simulink model "newFS_safetyTests"  (R2019a)
settings: Solver=FixedStepAuto  StartTime=0.0  StopTime=70  FixedStep=0.01  RelTol=1e-3
libraries: simulink x2, autolibshared x2, vehdynlibsteering x2, autolibutils x2, eeGeneralControl x1
settings Model: Creator=ckreienk  LastModifiedBy=ckreienk

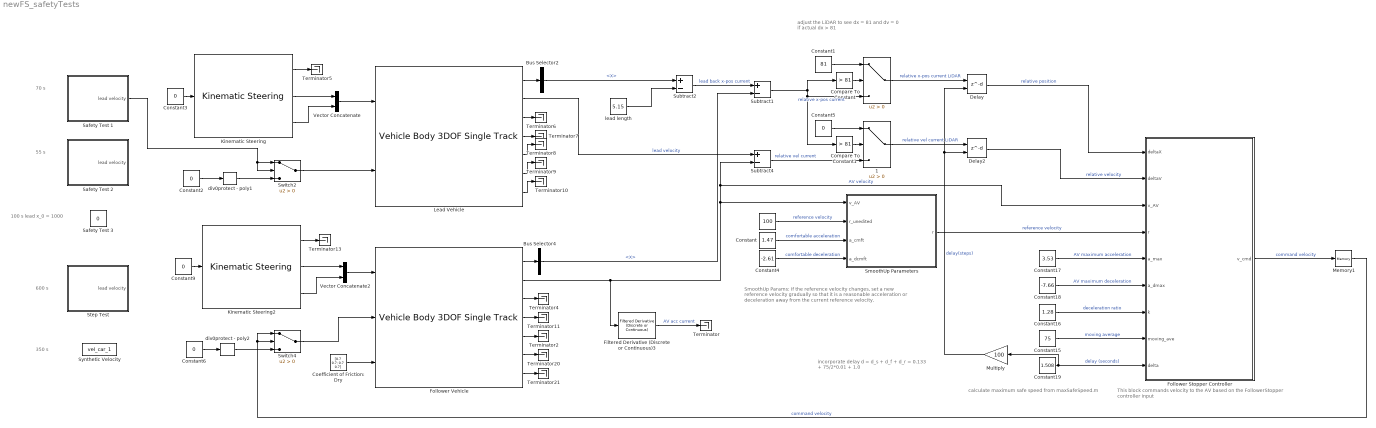
== system newFS_safetyTests ==
  note: adjust the LiDAR to see
      | dx = 81 and dv = 0
      | if actual dx > 81
  note: incorporate delay
      | d = d_s + d_f + d_r
      | = 0.133 + 75/2*0.01 + 1.0
  note: SmoothUp Params:
      | If the reference velocity changes,
      | set a new reference velocity gradually
      | so that it is a reasonable acceleration
      | or deceleration away from the current
      | reference velocity.
  note: This block commands velocity to the AV based
      | on the FollowerStopper controller input
  note: calculate maximum safe speed
      | from maxSafeSpeed.m
  note: 55 s
  note: 100 s
      | lead x_0 = 1000
  note: 600 s
  note: 70 s
  note: 350 s
  " " : Switch  Criteria=u2 > Threshold
  "  " : Constant  Value=100
  " 1" : Switch  Criteria=u2 > Threshold
  Bus Selector2 : BusSelector  OutputSignals=InertFrm.Geom.Disp.X
  Bus Selector4 : BusSelector  OutputSignals=InertFrm.Geom.Disp.X
  Coefficient of Friction: Dry : Constant  Value=[0.7 0.7; 0.7 0.7]
  Compare To Constant : simulink/Logic and Bit Operations/Compare To Constant  relop=>  const=81  OutDataTypeStr=boolean
  Compare To Constant1 : simulink/Logic and Bit Operations/Compare To Constant  relop=>  const=81  OutDataTypeStr=boolean
  Constant : Constant  Value=1.47
  Constant1 : Constant  Value=81
  Constant15 : Constant  Value=75
  Constant16 : Constant  Value=1.28
  Constant17 : Constant  Value=3.53
  Constant18 : Constant  Value=-7.66
  Constant19 : Constant  Value=1.508
  Constant{2..3,5..6,9} (5 alike) : Constant  Value=0
  Constant4 : Constant  Value=-2.61
  Delay : Delay  DelayLengthSource=Input port  DelayLength=183
      settings: InputPortMap=u0,p1
  Delay2 : Delay  DelayLengthSource=Input port  DelayLength=183
      settings: InputPortMap=u0,p1
  Filtered Derivative (Discrete or Continuous)3 : eeGeneralControl/Filtered Derivative (Discrete or Continuous)  K=1  T=0.1  B=20  A=-20  minRatio=10  Ts=-1
      settings: SourceProductName=Simscape Electrical  SourceProductBaseCode=PS
  Follower Stopper Controller : Subsystem
  Follower Vehicle : autolibshared/Vehicle Body 3DOF Single Track  trackMode=Dual  inputMode=External longitudinal velocity  frontSteerMode=on  rearSteerMode=off  windMode=off  muMode=on  extFMode=off  extMMode=off  extXo=off  extpsio=off  extxdoto=off  extro=off  extYo=off  extTamb=off  extydoto=off  aMode=2  NF=2  NR=2  m=2000  a=1.4  b=1.6  h=0.35  X_o=0  xdot_o=0  CalphaMode=off  sigmaMode=on  d=0  w=[1.4,1.4]  Cy_f=12e3  Cy_r=11e3  sigma_f=.1  sigma_r=.1  alpha_f_brk=[-.1 .1]  Cy_f_data=[-9e3 9e3]  alpha_r_brk=[-.1 .1]  Cy_r_data=[-9e3 9e3]  Y_o=0  ydot_o=0  Izz=4000  psi_o=0  r_o=0  Af=2  Cd=.3  Cl=.1  Cpm=.1  beta_w=[0:0.01:0.3]  Cs=[0:0.03:0.9]  Cym=[0:0.01:0.3]  Pabs=101325  Tair=273  g=9.81  mu=1  xdot_tol=.01  Fznom=5000  Fxtire_sat=7e4  Fytire_sat=7e4  longOff=0  latOff=0  vertOff=0  wrapAng=off
      settings: SourceProductName=Powertrain Blockset  SourceProductBaseCode=PW
  Kinematic Steering : vehdynlibsteering/Kinematic Steering  StrgType=Ackerman  StrgRatioType=Constant  Loc=Front  NrmlFctr=0.01  TrckWdth=1  WhlBase=1.524  Db=0  StrgRng=1.25*pi  StrgAngBpts="[-6.2832   -5.0265   -3.7699   -2.5133   -1.2566         0    1.2566    2.5133    3.7699    5.0265    6.2832]"  StrgRatioTbl=|  StrgRatio=100  StrgArmLngth=0.1  RckCsLngth=0.5  TieRodLngth=0.248  D=0.2  PnnRadius=0.0057  PnnRadiusTbl="[0.0055    0.0055    0.0056    0.0057    0.0058    0.0057    0.0057    0.0057    0.0056    0.0055    0.0055]"  RodLngth=0.1  ParaArmLngth=0.9  aMode=2
      | [13.5000   13.3750   13.2500   13.1250   13.0000   13.0000   13.0000   13.1250   13.2500   13.3750   13.5000
      | ]
      settings: SourceProductName=Vehicle Dynamics Blockset
  Kinematic Steering2 : vehdynlibsteering/Kinematic Steering  StrgType=Ackerman  StrgRatioType=Constant  Loc=Front  NrmlFctr=0.01  TrckWdth=1  WhlBase=1.524  Db=0  StrgRng=1.25*pi  StrgAngBpts="[-6.2832   -5.0265   -3.7699   -2.5133   -1.2566         0    1.2566    2.5133    3.7699    5.0265    6.2832]"  StrgRatioTbl=|  StrgRatio=100  StrgArmLngth=0.1  RckCsLngth=0.5  TieRodLngth=0.248  D=0.2  PnnRadius=0.0057  PnnRadiusTbl="[0.0055    0.0055    0.0056    0.0057    0.0058    0.0057    0.0057    0.0057    0.0056    0.0055    0.0055]"  RodLngth=0.1  ParaArmLngth=0.9  aMode=2
      | [13.5000   13.3750   13.2500   13.1250   13.0000   13.0000   13.0000   13.1250   13.2500   13.3750   13.5000
      | ]
      settings: SourceProductName=Vehicle Dynamics Blockset
  Lead Vehicle : autolibshared/Vehicle Body 3DOF Single Track  trackMode=Dual  inputMode=External longitudinal velocity  frontSteerMode=on  rearSteerMode=off  windMode=off  muMode=off  extFMode=off  extMMode=off  extXo=off  extpsio=off  extxdoto=off  extro=off  extYo=off  extTamb=off  extydoto=off  aMode=2  NF=2  NR=2  m=2000  a=1.4  b=1.6  h=0.35  X_o=10  xdot_o=0  CalphaMode=off  sigmaMode=on  d=0  w=[1.4,1.4]  Cy_f=12e3  Cy_r=11e3  sigma_f=.1  sigma_r=.1  alpha_f_brk=[-.1 .1]  Cy_f_data=[-9e3 9e3]  alpha_r_brk=[-.1 .1]  Cy_r_data=[-9e3 9e3]  Y_o=0  ydot_o=0  Izz=4000  psi_o=0  r_o=0  Af=2  Cd=.3  Cl=.1  Cpm=.1  beta_w=[0:0.01:0.3]  Cs=[0:0.03:0.9]  Cym=[0:0.01:0.3]  Pabs=101325  Tair=273  g=9.81  mu=1  xdot_tol=.01  Fznom=5000  Fxtire_sat=7e4  Fytire_sat=7e4  longOff=0  latOff=0  vertOff=0  wrapAng=off
      settings: SourceProductName=Powertrain Blockset  SourceProductBaseCode=PW
  Memory1 : Memory
  Multiply : Gain  Gain=100
  Safety Test 1 : Subsystem
  Safety Test 2 : Subsystem
  Safety Test 3 : Constant  Value=0
  SmoothUp Parameters : MATLAB Function  TreatAsAtomicUnit=on
  Step Test : Subsystem
  Subtract1 : Sum  Inputs=+-
  Subtract2 : Sum  Inputs=+-
  Subtract4 : Sum  Inputs=+-
  Switch2 : Switch  Criteria=u2 > Threshold
  Switch4 : Switch  Criteria=u2 > Threshold
  Synthetic Velocity : FromWorkspace  VariableName=vel_car_1
  Terminator{,2,4..11,13,20..21} (13 alike) : Terminator
  Vector Concatenate : Concatenate
  Vector Concatenate2 : Concatenate
  div0protect - poly1 : autolibutils/div0protect - poly  thresh=1e-3  aMode=2
      settings: SourceProductName=Powertrain Blockset  SourceProductBaseCode=PW
  div0protect - poly2 : autolibutils/div0protect - poly  thresh=1e-3  aMode=2
      settings: SourceProductName=Powertrain Blockset  SourceProductBaseCode=PW
  lead length : Constant  Value=5.15
  wires:
  Kinematic Steering2/2 -> Vector Concatenate2/1
  Subtract2/1 -> Subtract1/1  "lead back x-pos current"
  Kinematic Steering2/3 -> Vector Concatenate2/2
  Bus Selector4/1 -> Subtract1/2  "<X>"
  lead length/1 -> Subtract2/2
  Follower Vehicle/5 -> Terminator2/1
  div0protect - poly2/1 -> Switch4/3
  Lead Vehicle/1 -> Bus Selector2/1
  Follower Vehicle/7 -> Terminator21/1
  Constant6/1 -> div0protect - poly2/1
  Kinematic Steering/3 -> Vector Concatenate/2
  Lead Vehicle/2 -> Subtract4/1  "lead velocity"
  Kinematic Steering/2 -> Vector Concatenate/1
  Follower Vehicle/3 -> Terminator4/1
  Follower Vehicle/6 -> Terminator20/1
  Switch2/1 -> Lead Vehicle/2
  Constant9/1 -> Kinematic Steering2/1
  Switch4/1 -> Follower Vehicle/2
  " "/1 -> Delay/1  "relative x-pos current LiDAR"
  Vector Concatenate/1 -> Lead Vehicle/1
  Lead Vehicle/5 -> Terminator8/1
  Follower Vehicle/1 -> Bus Selector4/1
  Lead Vehicle/4 -> Terminator7/1
  Coefficient of Friction: Dry/1 -> Follower Vehicle/3
  Constant1/1 -> " "/1
  Subtract1/1 -> Compare To Constant/1, Compare To Constant1/1, " "/3  "relative x-pos current"
  Kinematic Steering2/1 -> Terminator13/1
  Bus Selector2/1 -> Subtract2/1  "<X>"
  Memory1/1 -> Switch4/1, Switch4/2  "command velocity"
  Constant2/1 -> div0protect - poly1/1
  Kinematic Steering/1 -> Terminator5/1
  Lead Vehicle/3 -> Terminator6/1
  div0protect - poly1/1 -> Switch2/3
  Follower Vehicle/4 -> Terminator11/1
  Compare To Constant/1 -> " "/2
  Lead Vehicle/7 -> Terminator10/1
  Constant3/1 -> Kinematic Steering/1
  Safety Test 1/1(lead velocity) -> Switch2/2, Switch2/1
  Follower Vehicle/2 -> Filtered Derivative (Discrete or Continuous)3/1, Subtract4/2, Follower Stopper Controller/3(v_AV), SmoothUp Parameters/1(v_AV)  "AV velocity"
  Lead Vehicle/6 -> Terminator9/1
  Vector Concatenate2/1 -> Follower Vehicle/1
  Delay/1 -> Follower Stopper Controller/1(deltaX)  "relative position"
  Delay2/1 -> Follower Stopper Controller/2(deltaV)  "relative velocity"
  Constant19/1 -> Follower Stopper Controller/9(delta), Multiply/1  "delay (seconds)"
  Constant16/1 -> Follower Stopper Controller/7(k)  "deceleration ratio"
  Constant17/1 -> Follower Stopper Controller/5(a_max)  "AV maximum acceleration"
  "  "/1 -> SmoothUp Parameters/2(r_unedited)  "reference velocity"
  Follower Stopper Controller/1(v_cmd) -> Memory1/1  "command velocity"
  Constant15/1 -> Follower Stopper Controller/8(moving_ave)  "moving average"
  Constant18/1 -> Follower Stopper Controller/6(a_dmax)  "AV maximum deceleration"
  SmoothUp Parameters/1(r) -> Follower Stopper Controller/4(r)  "reference velocity"
  Constant/1 -> SmoothUp Parameters/3(a_cmft)  "comfortable acceleration"
  Constant4/1 -> SmoothUp Parameters/4(a_dcmft)  "comfortable deceleration"
  Multiply/1 -> Delay/2, Delay2/2  "delay(steps)"
  Compare To Constant1/1 -> " 1"/2
  Constant5/1 -> " 1"/1
  Subtract4/1 -> " 1"/3  "relative vel current"
  " 1"/1 -> Delay2/1  "relative vel current LiDAR"
  Filtered Derivative (Discrete or Continuous)3/1 -> Terminator/1  "AV acc current"

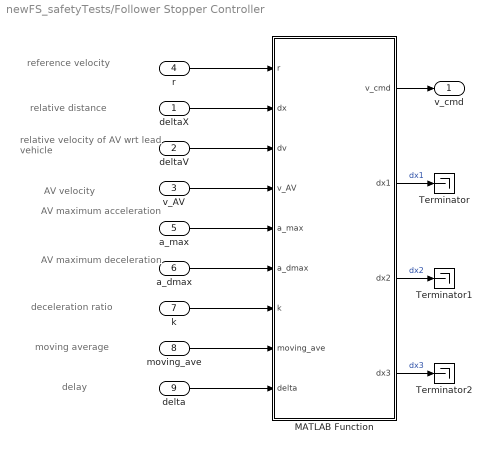
== system newFS_safetyTests/Follower Stopper Controller ==
  note: relative distance
  note: reference velocity
  note: AV velocity
  note: relative velocity of
      | AV wrt lead vehicle
  note: AV maximum
      | acceleration
  note: AV maximum
      | deceleration
  note: deceleration ratio
  note: moving average
  note: delay
  deltaX : Inport
  deltaV : Inport  Port=2
  v_AV : Inport  Port=3
  r : Inport  Port=4
  a_max : Inport  Port=5
  a_dmax : Inport  Port=6
  k : Inport  Port=7
  moving_ave : Inport  Port=8
  delta : Inport  Port=9
  MATLAB Function : MATLAB Function  TreatAsAtomicUnit=on
  Terminator : Terminator
  Terminator1 : Terminator
  Terminator2 : Terminator
  v_cmd : Outport
  wires:
  r/1 -> MATLAB Function/1(r)
  v_AV/1 -> MATLAB Function/4(v_AV)
  MATLAB Function/1(v_cmd) -> v_cmd/1
  deltaV/1 -> MATLAB Function/3(dv)
  deltaX/1 -> MATLAB Function/2(dx)
  moving_ave/1 -> MATLAB Function/8(moving_ave)
  a_max/1 -> MATLAB Function/5(a_max)
  a_dmax/1 -> MATLAB Function/6(a_dmax)
  k/1 -> MATLAB Function/7(k)
  delta/1 -> MATLAB Function/9(delta)
  MATLAB Function/2(dx1) -> Terminator/1  "dx1"
  MATLAB Function/3(dx2) -> Terminator1/1  "dx2"
  MATLAB Function/4(dx3) -> Terminator2/1  "dx3"

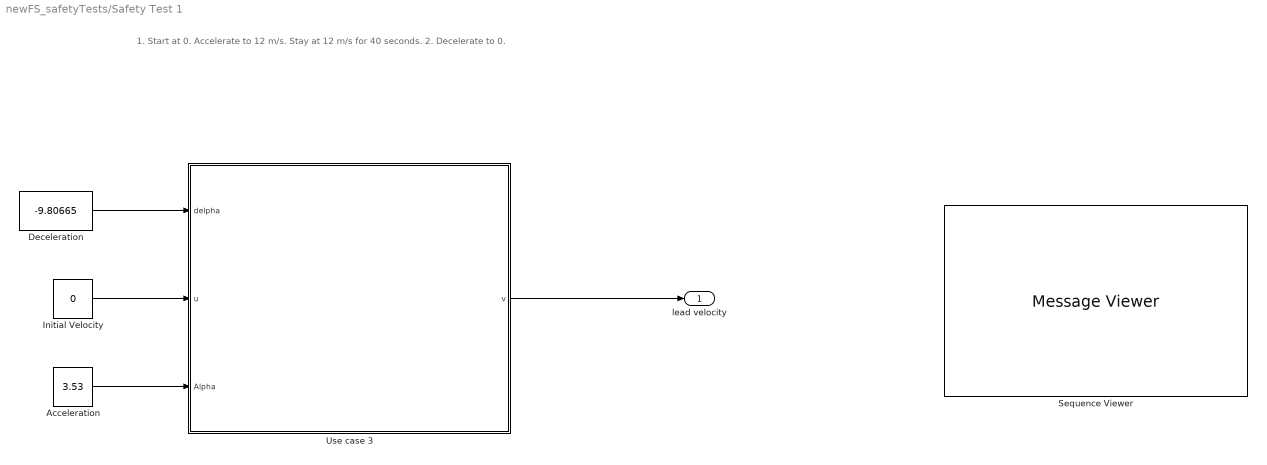
== system newFS_safetyTests/Safety Test 1 ==
  note: 1. Start at 0. Accelerate to 12 m/s. Stay at 12 m/s for 40 seconds.
      | 2. Decelerate to 0.
  Acceleration : Constant  Value=3.53
  Deceleration : Constant  Value=-9.80665
  Initial Velocity : Constant  Value=0
  Sequence Viewer : MessageViewer
  Use case 3 : Stateflow chart  TreatAsAtomicUnit=on
  lead velocity : Outport
  wires:
  Acceleration/1 -> Use case 3/3(Alpha)
  Initial Velocity/1 -> Use case 3/2(u)
  Deceleration/1 -> Use case 3/1(delpha)
  Use case 3/1(v) -> lead velocity/1

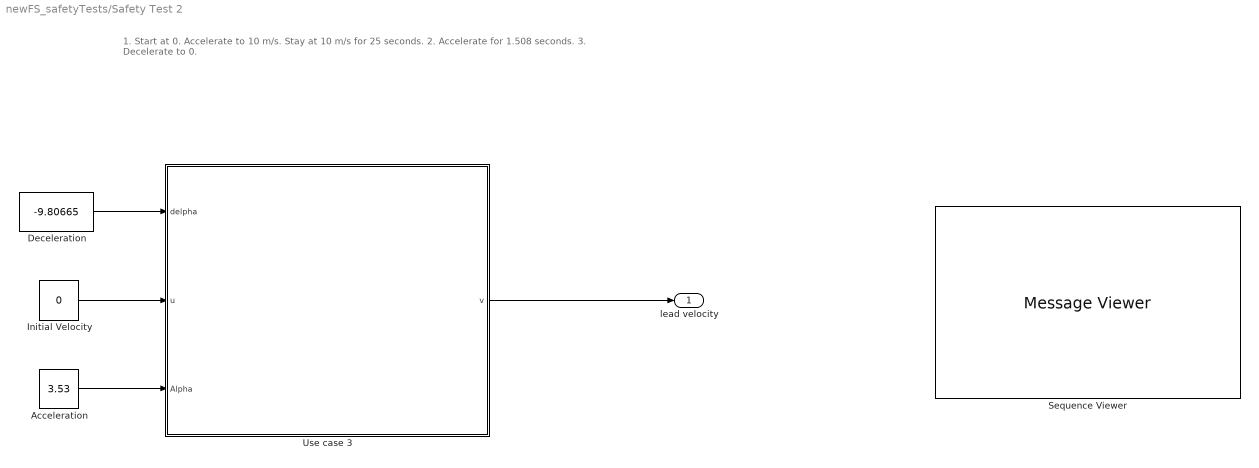
== system newFS_safetyTests/Safety Test 2 ==
  note: 1. Start at 0. Accelerate to 10 m/s. Stay at 10 m/s for 25 seconds.
      | 2. Accelerate for 1.508 seconds.
      | 3. Decelerate to 0.
  Acceleration : Constant  Value=3.53
  Deceleration : Constant  Value=-9.80665
  Initial Velocity : Constant  Value=0
  Sequence Viewer : MessageViewer
  Use case 3 : Stateflow chart  TreatAsAtomicUnit=on
  lead velocity : Outport
  wires:
  Use case 3/1(v) -> lead velocity/1
  Deceleration/1 -> Use case 3/1(delpha)
  Initial Velocity/1 -> Use case 3/2(u)
  Acceleration/1 -> Use case 3/3(Alpha)

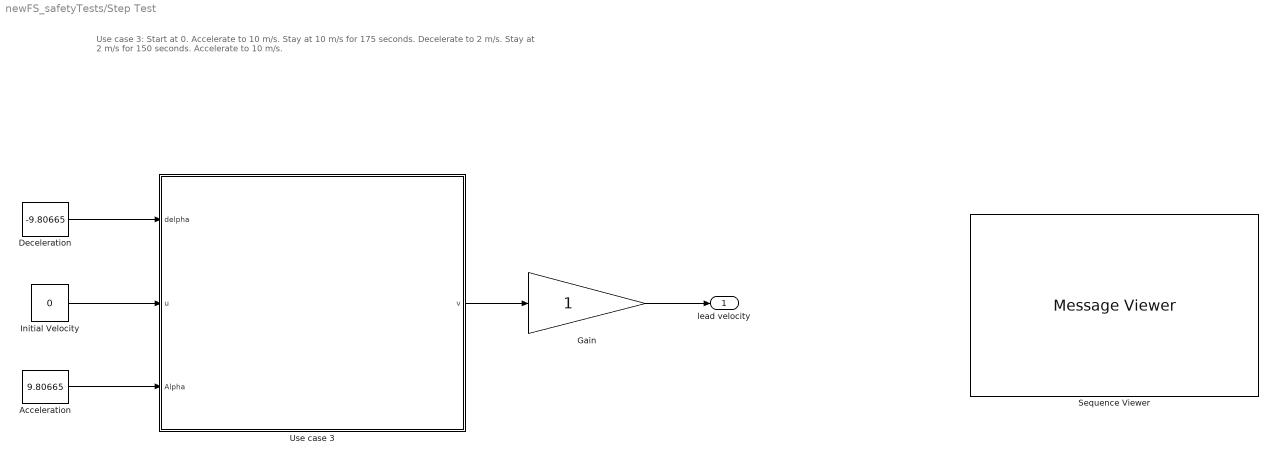
== system newFS_safetyTests/Step Test ==
  note: Use case 3:
      | Start at 0. Accelerate to 10 m/s. Stay at 10 m/s for 175 seconds.
      | Decelerate to 2 m/s. Stay at 2 m/s for 150 seconds.
      | Accelerate to 10 m/s.
  Acceleration : Constant  Value=9.80665
  Deceleration : Constant  Value=-9.80665
  Gain : Gain
  Initial Velocity : Constant  Value=0
  Sequence Viewer : MessageViewer
  Use case 3 : Stateflow chart  TreatAsAtomicUnit=on
  lead velocity : Outport
  wires:
  Use case 3/1(v) -> Gain/1
  Acceleration/1 -> Use case 3/3(Alpha)
  Initial Velocity/1 -> Use case 3/2(u)
  Deceleration/1 -> Use case 3/1(delpha)
  Gain/1 -> lead velocity/1

== stateflow chart newFS_safetyTests/Safety Test 2/Use case 3 ==
  state Hold
    entry: u2 = v;
    during: v = u2;
    exit:
    note: HOLD STATE
  state Accelerate
    entry: entryState = 1; v = 0;
    during: v = getNewVaccel(v, Alpha)
    exit:  nextState = entryState + 1;
    note: STATE 1
  state Accelerate1
    entry: entryState = nextState; v = u2;
    during: v = getNewVaccel(v, Alpha);
    exit: nextState = entryState + 1;
    note: STATE 2
  state Decelerate
    entry: entryState = nextState; v = u2;
    during: v = getNewVdecel(v,delpha);
    exit: nextState = entryState + 1;
    note: STATE 3
  state Hold1
    entry:
    during: v = 0;
    exit:
  state zero
    entry: v = 0;
    during:v = 0;
    note: STATE 4
  (default) -> Accelerate
  Hold -> Accelerate1 : [after(25, sec)]
  Accelerate -> Hold : [v>=10 ]
  Accelerate1 -> Decelerate : [after(1.508, sec)]
  Decelerate -> Hold1 : [v==0]
  Hold1 -> zero
  data: init_velocity function_input; deceleration function_input; new_vel function_output; init_velocity function_input; acceleration function_input; new_vel function_output; delpha input; u input; Alpha input; v output =0; u2 local =0; entryState local =0; nextState local =0
  function new_vel = getNewVdecel(init_velocity, deceleration):
    | function new_vel = getNewVdecel(init_velocity, deceleration)
    | 
    | new_vel = init_velocity - abs(deceleration*0.01);
    | new_vel = max(new_vel,0);
    | 
    | end
  function new_vel = getNewVaccel(init_velocity, acceleration):
    | function new_vel = getNewVaccel(init_velocity, acceleration)
    | 
    | new_vel = init_velocity + (acceleration*0.01);
    | 
    | end

== matlab function newFS_safetyTests/Follower Stopper Controller/MATLAB Function ==
  settings: updateMethod=DISCRETE
  data: r input; dx input; dv input; v_cmd output; v_AV input; a_max input; a_dmax input; k input; moving_ave input; delta input; dx1 output; dx2 output; dx3 output
function [v_cmd, dx1, dx2, dx3] = fcn(r,dx,dv,v_AV,...
    a_max, a_dmax, k, moving_ave, delta)

%#codegen
% Safety controller, based on quadratic bands.
% Input: r = desired velocity (from other models)
%          dx = estimate of gap to vehicle ahead
%          dv = estimate of time derivative of dx (= velocity difference)
%        v_AV = velocity of AV
%      a_cmft = comfortable acceleration
%      a_dmax = maximum AV deceleration
%           k = ratio between maximum lead deceleration and a_dmax
%  moving_ave = number of v_cmd data points of which to take the average
% Out:  v_cmd = actual velocity commanded (always v_cmd<=r)
%
% Controller-specific parameters

% Lead vehicle velocity
v_lead = v_AV+dv; % velocity of lead vehicle
v_lead = max(v_lead,0); % lead vehicle cannot go backwards
v = min(r,v_lead); % safety velocity cannot exceed desired velocity r

% Relative distance parameters
deltaVSStar = max(1/(2*k*a_dmax)*(v_lead^2-k*v_AV^2),0);
dx1 = 1+deltaVSStar + v_AV*(1-a_max/a_dmax)*delta + a_max/2*(1-a_max/a_dmax)*delta^2;
%dx1 = 1+deltaVSStar + v_AV*delta;
dx2 = dx1 + 2*v_AV*delta;
dx3 = 2*dx2-dx1;

% Actual commanded velocity
new_cmd = double((dx<=dx1).*(0))+...
    (dx1<dx&dx<=dx2).*(v*(dx-dx1)/(dx2-dx1))+...
    (dx2<dx&dx<=dx3).*(v + (r-v)*(dx-dx2)/(dx3-dx2))+...
    (dx3<dx).*(r);

% Take moving average of last moving_ave number of values
persistent moving_array
if isempty(moving_array)
    moving_array=zeros(1,moving_ave);
end
moving_array = [moving_array(2:moving_ave) new_cmd];
new_cmd_ave = mean(moving_array,'all');

% Make sure the moving average is within the maximum braking and maximum
% acceleration of the Ford Hybrid Escape
dt = 0.01;
possibleAcc = v_AV + a_max*dt;
possibleDec = v_AV + a_dmax*dt;
v_cmd = min(max(new_cmd_ave,possibleDec),possibleAcc);

== stateflow chart newFS_safetyTests/Safety Test 1/Use case 3 ==
  state zero
    entry: v = 0;
    during:v = 0;
    note: STATE 4
  state Hold
    entry: u2 = v;
    during: v = u2;
    exit:
    note: HOLD STATE
  state AccelerateTo60_init
    entry: entryState = 1; v = 0;
    during: v = getNewVaccel(v, Alpha)
    exit:  nextState = entryState + 1;
    note: STATE 1
  state Hold1
    entry:
    during: v = 0;
    exit:
  state Accelerate
    entry: entryState = nextState; v = u2;
    during: v = getNewVdecel(v,delpha);
    exit: nextState = entryState + 1;
    note: STATE 2
  Hold1 -> zero
  (default) -> AccelerateTo60_init
  Hold -> Accelerate : [after(40, sec)]
  AccelerateTo60_init -> Hold : [v>=12 ]
  Accelerate -> Hold1 : [v==0]
  data: init_velocity function_input; deceleration function_input; new_vel function_output; init_velocity function_input; acceleration function_input; new_vel function_output; delpha input; u input; Alpha input; v output =0; u2 local =0; entryState local =0; nextState local =0
  function new_vel = getNewVdecel(init_velocity, deceleration):
    | function new_vel = getNewVdecel(init_velocity, deceleration)
    | 
    | new_vel = init_velocity - abs(deceleration*0.01);
    | new_vel = max(new_vel,0);
    | 
    | end
  function new_vel = getNewVaccel(init_velocity, acceleration):
    | function new_vel = getNewVaccel(init_velocity, acceleration)
    | 
    | new_vel = init_velocity + (acceleration*0.01);
    | 
    | end

== stateflow chart newFS_safetyTests/Step Test/Use case 3 ==
  note: Use case 3:
      | Start at 0. Accelerate to 20mph. Stay at 20mph for 30 seconds.
      | Accelerate the speed to increase it by 5mph. Stay for 30 seconds.
      | If speed reaches 60mph, decelerate to 0.
  state zero
    entry: v = 0;
    during:v = 0;
    note: STATE 4
  state Hold
    entry: u2 = v;
    during: v = u2;
    exit:
    note: HOLD STATE
  state AccelerateTo60_init
    entry: entryState = 1; v = 0;
    during: v = getNewVaccel(v, Alpha)
    exit:  nextState = entryState + 1;
    note: STATE 1
  state Hold1
    entry: u2 = v;
    during: v = u2;
    exit:
    note: HOLD STATE
  state Accelerate
    entry: entryState = nextState; v = u2;
    during: v = getNewVdecel(v,delpha);
    exit: nextState = entryState + 1;
    note: STATE 2
  state Hold2
    entry: u2 = v;
    during: v = u2;
    exit:
    note: HOLD STATE
  state AccelerateTo60_init1
    entry: entryState = 1; v = 3;
    during: v = getNewVaccel(v, Alpha)
    exit:  nextState = entryState + 1;
    note: STATE 1
  state Accelerate1
    entry: entryState = nextState; v = u2;
    during: v = getNewVdecel(v,delpha);
    exit: nextState = entryState + 1;
    note: STATE 2
  state Hold3
    entry:
    during: v = 0;
    exit:
  Hold3 -> zero : [v==0]
  (default) -> AccelerateTo60_init
  Hold -> Accelerate : [after(175, sec)]
  AccelerateTo60_init -> Hold : [v>=10]
  Accelerate -> Hold1 : [v<=2]
  Hold1 -> AccelerateTo60_init1 : [after(150, sec)]
  Hold2 -> Accelerate1 : [after(300, sec)]
  AccelerateTo60_init1 -> Hold2 : [v>=10 ]
  Accelerate1 -> Hold3 : [v==0]
  data: init_velocity function_input; deceleration function_input; new_vel function_output; init_velocity function_input; acceleration function_input; new_vel function_output; delpha input; u input; Alpha input; v output =0; u2 local =0; entryState local =0; nextState local =0
  function new_vel = getNewVdecel(init_velocity, deceleration):
    | function new_vel = getNewVdecel(init_velocity, deceleration)
    | 
    | new_vel = init_velocity - abs(deceleration*0.01);
    | new_vel = max(new_vel,0);
    | 
    | end
  function new_vel = getNewVaccel(init_velocity, acceleration):
    | function new_vel = getNewVaccel(init_velocity, acceleration)
    | 
    | new_vel = init_velocity + (acceleration*0.01);
    | new_vel = min(new_vel,10);
    | 
    | end

== matlab function newFS_safetyTests/SmoothUp Parameters ==
  settings: updateMethod=DISCRETE
  data: v_AV input; r_unedited input; r output; a_cmft input; a_dcmft input
function r = fcn(v_AV,r_unedited,a_cmft,a_dcmft)
% #codegen
persistent y

if isempty(y)
    y=v_AV;
end

dt=0.01;
if( y > r_unedited + a_cmft*dt)
    y = max(r_unedited,y - abs(a_dcmft)*dt);
elseif( y < r_unedited - abs(a_dcmft)*dt)
    y = min(r_unedited,y + a_cmft*dt);
else
    y = r_unedited;
end

r = y;
